simulink model "PMSM_SMC_C"  (R2022b)
settings: Solver=ode23tb  StartTime=0.0  StopTime=1  FixedStep=Ts  RelTol=1e-4  EnableMultiTasking=on
InitFcn:
  | Ts = 10e-6;
  | 
  | R = 2.875;
  | Ld = 8.2e-3;
  | Lq = 8.2e-3;
  | Pn = 4;
  | flux = 0.175;
  | alpha1=15;
  | alpha2=9;
  | e=0.0005;
  | B = 0;
  | J = 0.003;
  | a=-(B/J);
  | b=(3*Pn*flux)/(2*J);
  | kq1=100;
  | kq2=80;
undefined symbols (not defined in the file): DiscIntNeverNeededParam, k1, k2
libraries: simulink x3, powerlib_extras x1, slpidlib x1, spsPermanentMagnetSynchronousMachineLib x1, spsUniversalBridgeLib x1, spsDCVoltageSourceLib x1, sps_lib x1
settings Model: Creator=SUN  LastModifiedBy=hl
settings SolverCC: ZeroCrossControl=DisableAll  AlgebraicLoopSolver=TrustRegion
settings DataIOCC: LimitDataPoints=on  SaveFormat=Array  SignalLoggingSaveFormat=ModelDataLogs  ReturnWorkspaceOutputs=off
settings OptimizationCC: ExpressionDepthLimit=2147483647  InitFltsAndDblsToZero=on  LifeSpan=inf
settings DebuggingCC: UnderspecifiedInitializationDetection=Classic  MergeDetectMultiDrivingBlocksExec=none  SolverPrmCheckMsg=warning  FcnCallInpInsideContextMsg=warning  UnconnectedInputMsg=warning  UnconnectedOutputMsg=warning  UnconnectedLineMsg=warning  StateNameClashWarn=warning  SFUnexpectedBacktrackingDiag=warning  SFNoUnconditionalDefaultTransitionDiag=warning  SFMachineParentedDataDiag=warning  ArithmeticOperatorsInVariantConditions=warning
settings HardwareCC: ProdBitPerPointer=32  ProdBitPerSizeT=32  ProdBitPerPtrDiffT=32  ProdLargestAtomicFloat=None  ProdIntDivRoundTo=Undefined  ProdEndianess=Unspecified  ProdWordSize=32  ProdHWDeviceType=32-bit Generic
settings ModelReferenceCC: EnableRefExpFcnMdlSchedulingChecks=on  PropagateSignalLabelsOutOfModel=off
settings SFSimCC: SimUseLocalCustomCode=off  CustomCodeUndefinedFunction=UseInterfaceOnly
settings RTWCC: RTWUseLocalCustomCode=off
settings CodeAppCC: StateflowObjectComments=on
settings GRTTargetCC: TargetLangStandard=C89/C90 (ANSI)  CombineOutputUpdateFcns=off  GRTInterface=on
settings ConfigComp: CovMetricSettings=dw  CovSaveCumulativeToWorkspaceVar=on  CovSaveSingleToWorkspaceVar=on  CovExternalEMLEnable=off  CovSFcnEnable=off
settings SimscapeCC: SimscapeNormalizeSystem=off

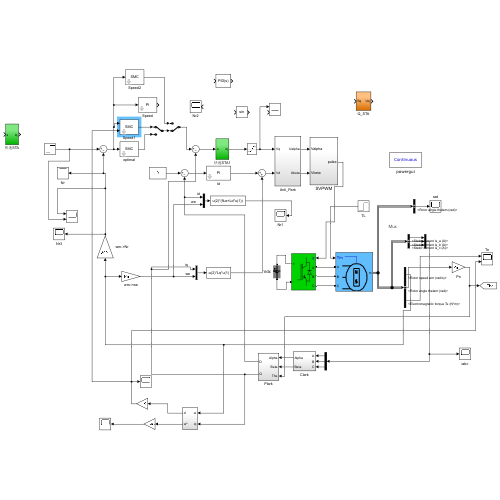
[thumbnail: Simulink's stored preview of the top-level diagram]
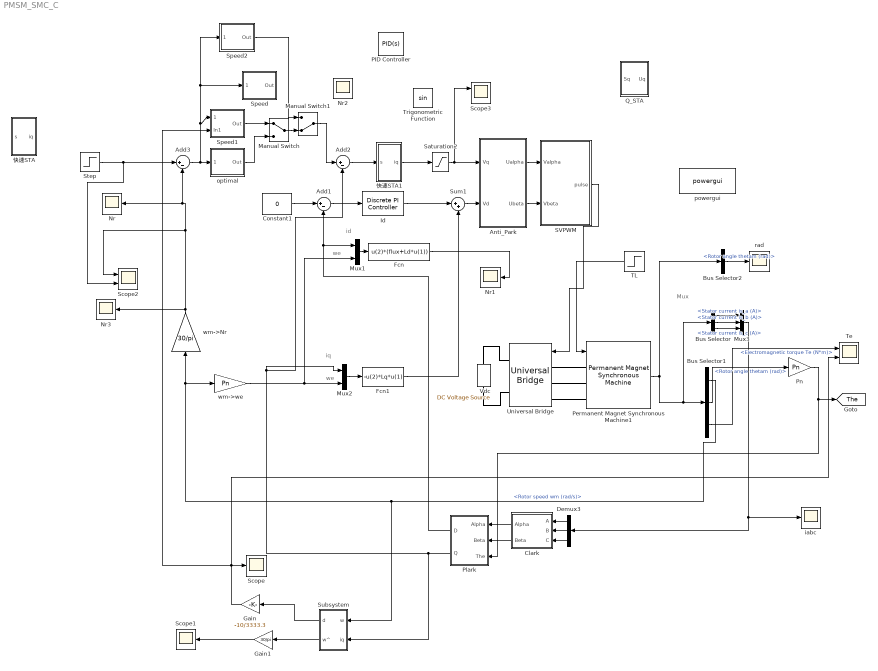
== system PMSM_SMC_C ==
  note: Mux
  note: iq
  note: we
  note: we
  note: id
  Add1 : Sum  Inputs=|+-
  Add2 : Sum  Inputs=|+-
  Add3 : Sum  Inputs=|+-
  Anti_Park : Subsystem
  Bus Selector : BusSelector  OutputSignals=Stator current is_a (A),Stator current is_b (A),Stator current is_c (A)
  Bus Selector1 : BusSelector  OutputSignals=Rotor speed wm (rad/s),Rotor angle thetam (rad),Electromagnetic torque Te (N*m)
  Bus Selector2 : BusSelector  OutputSignals=Rotor angle thetam (rad)
  Clark : Subsystem
  Constant1 : Constant  Value=0
  Demux3 : Demux  Outputs=3
  Fcn : Fcn  Expr=u(2)*(flux+Ld*u(1))
  Fcn1 : Fcn  Expr=-u(2)*Lq*u(1)
  Gain : Gain  Gain=-10/3333.3
  Gain1 : Gain  Gain=30/pi
  Id : powerlib_extras/Discrete  Control Blocks/Discrete PI Controller  Kp=Ld*2000  Ki=R*2000  Par_Limits=[311*0.9*sqrt(1/3) -311*0.9*sqrt(1/3)]  Init=0  Ts=Ts
  Manual Switch : ManualSwitch
  Manual Switch1 : ManualSwitch  CurrentSetting=0
  Mux1 : Mux  Inputs=2
  Mux2 : Mux  Inputs=2
  Mux3 : Mux  Inputs=3
  Nr{,1..3} (4 alike) : Scope
  PID Controller : slpidlib/PID Controller  Controller=PID  Form=Parallel  TimeDomain=Continuous-time  UseExternalTs=off  SampleTime=-1  IntegratorMethod=Forward Euler  FilterMethod=Forward Euler  ControllerParametersSource=internal  P=60  I=10  UseKiTs=off  D=0  N=100  UseFilter=on  TunerSelectOption=Transfer Function Based (PID Tuner App)  InitialConditionSource=internal  InitialConditionForIntegrator=0  InitialConditionForFilter=0  DifferentiatorICPrevScaledInput=0  ExternalReset=none  TrackingMode=off  Kt=1  LimitOutput=off  SatLimitsSource=internal  UpperSaturationLimit=inf  LowerSaturationLimit=-inf  LinearizeAsGain=on  AntiWindupMode=none  Kb=1  LimitIntegrator=off  UpperIntegratorSaturationLimit=inf  LowerIntegratorSaturationLimit=-inf  POutMin=[]  POutMax=[]  IOutMin=[]  IOutMax=[]  DOutMin=[]  DOutMax=[]  NOutMin=[]  NOutMax=[]  SumOutMin=[]  SumOutMax=[]  SaturationOutMin=[]  SaturationOutMax=[]  PParamMin=[]  PParamMax=[]  IParamMin=[]  IParamMax=[]  DParamMin=[]  DParamMax=[]  NParamMin=[]  NParamMax=[]  KbParamMin=[]  KbParamMax=[]  KtParamMin=[]  KtParamMax=[]  KbOutMin=[]  KbOutMax=[]  KtOutMin=[]  KtOutMax=[]  IntegratorOutMin=[]  IntegratorOutMax=[]  FilterOutMin=[]  FilterOutMax=[]  SumI1OutMin=[]  SumI1OutMax=[]  SumI2OutMin=[]  SumI2OutMax=[]  SumI3OutMin=[]  SumI3OutMax=[]  SumI4OutMin=[]  SumI4OutMax=[]  SumDOutMin=[]  SumDOutMax=[]  DifferentiatorOutMin=[]  DifferentiatorOutMax=[]  FilterDiffOutCoefMin=[]  FilterDiffOutCoefMax=[]  ReciprocalOutMin=[]  ReciprocalOutMax=[]  SumDenOutMin=[]  SumDenOutMax=[]  SumNumOutMin=[]  SumNumOutMax=[]  DivideOutMin=[]  DivideOutMax=[]  UdiffTsProdOutMin=[]  UdiffTsProdOutMax=[]  NTsProdOutMin=[]  NTsProdOutMax=[]  UintegralTsProdOutMin=[]  UintegralTsProdOutMax=[]  UngainTsProdOutMin=[]  UngainTsProdOutMax=[]  ClampingZeroOutDataTypeStr=Inherit: Inherit via back propagation  ClampingZeroOutMin=[]  ClampingZeroOutMax=[]  FilterDenConstantOutDataTypeStr=Inherit: Inherit via back propagation  FilterDenConstantOutMin=[]  FilterDenConstantOutMax=[]  PCopyOutDataTypeStr=Inherit: Inherit via back propagation  PCopyOutMin=[]  PCopyOutMax=[]  NCopyOutDataTypeStr=Inherit: Inherit via back propagation  NCopyOutMin=[]  NCopyOutMax=[]  IntegratorContinuousStateAttributes=''  IntegratorStateMustResolveToSignalObject=off  IntegratorRTWStateStorageClass=Auto  FilterContinuousStateAttributes=''  FilterStateMustResolveToSignalObject=off  FilterRTWStateStorageClass=Auto  ParallelPVariant=InternalParameters  IdealPVariant=Disabled  IVariant=InternalParameters  DVariant=InternalParameters  IntegratorVariant=Continuous  SatVariant=Disabled  AWVariant=Passthrough  PCopyVariant=Disabled  TRVariant=Disabled  FdbkBlocksVariant=Forward  IdealPFdbkVariant=Disabled  SatFdbkVariant=Disabled  DerivativeFilterVariant=ContFilter  NVariant=InternalParameters  NCopyVariant=Disabled  FilterICVariant=InternalICsFilter  IntegratorICVariant=InternalICs  ExternalResetVariant=Disabled  TRSumVariant=Passthrough  SumFdbkVariant=Disabled  SumVariant=Sum_PID  TsampFilterVariant=InternalTs  TsampNgainVariant=Passthrough  TsampIntegralVariant=Passthrough  ExternalSaturationOutDataTypeStr=Inherit: Same as second input
  Permanent Magnet Synchronous Machine1 : spsPermanentMagnetSynchronousMachineLib/Permanent Magnet Synchronous Machine  NbPhases=3  FluxDistribution=Sinusoidal  RotorType=Salient-pole  MechanicalLoad=Torque Tm  PresetModel=No  ShowDetailedParameters=on  MeasurementBus=off  Resistance=2.875  Inductance=8.5e-3  dqInductances=[8.5e-3,8.5e-3]  La=0.000835  MachineConstant=Flux linkage established by magnets (V.s)  Flux=0.175  VoltageCst=126.966  TorqueCst=1.05  Flat=120  Mechanical=[0.003 0.008 4 0]  PolePairs=3  InitialConditions=[0,0, 0,0]  InitialConditions5ph=[0 0 0 0 0 0]  RefAngle=Aligned with phase A axis (original Park)  IterativeDiscreteModel=Trapezoidal non iterative  TsBlock=-1  TsPowergui=0
  Plark : Subsystem
  Pn : Gain  Gain=Pn
  Q_STA : Subsystem
  SVPWM : Subsystem
  Saturation2 : Saturate  UpperLimit=380  LowerLimit=-400  SampleTime=Ts
  Scope : Scope
  Scope1 : Scope
  Scope2 : Scope  NumInputPorts=2
  Scope3 : Scope  NumInputPorts=2
  Speed : Subsystem  AncestorBlock=|  DialogController=POWERSYS.PowerSysDialog  mask(Discrete PI Controller){Kpw=0.14, Kiw=0.14*50, Ba=0.013, Par_Limits=[30 -30], Init=0, Ts=Ts}
      | powerlib_extras/Discrete 
      | Control Blocks/Discrete
      | PI Controller
      mask prompts: Kpw "Proportional gain (Kp):"; Kiw "Integral gain (Ki):"; Ba "feedback gain (Ba)"; Par_Limits "Output limits: [ Upper   Lower ]"; Init "Output initial value:"; Ts "Sample time:"
      mask help: This block implements a discrete PI controller.
      mask init:
      | UpperLimit=Par_Limits(1);
      | LowerLimit=Par_Limits(2);
      | power_initmask();
      settings: LibrarySourceBlock=|
      | powerlib_extras/Discrete
      | Control Blocks/Discrete
      | PI Controller
      mask Help: This block is part of a subset of blocks in the Extras library that does not have documentation associated with it, other than the block mask description.
      mask Display: disp('PI');
  Speed1 : Subsystem  AncestorBlock=|  DialogController=POWERSYS.PowerSysDialog  mask(Discrete PI Controller){C=600, Mu=200, q=300, Par_Limits=[30 -30], Init=0, Ts=Ts}
      | powerlib_extras/Discrete 
      | Control Blocks/Discrete
      | PI Controller
      mask prompts: C "Gain (c):"; Mu "Gain (Mu):"; q "Gain (q)"; Par_Limits "Output limits: [ Upper   Lower ]"; Init "Output initial value:"; Ts "Sample time:"
      mask help: This block implements a discrete PI controller.
      mask init:
      | UpperLimit=Par_Limits(1);
      | LowerLimit=Par_Limits(2);
      | power_initmask();
      settings: LibrarySourceBlock=|
      | powerlib_extras/Discrete
      | Control Blocks/Discrete
      | PI Controller
      mask Help: This block is part of a subset of blocks in the Extras library that does not have documentation associated with it, other than the block mask description.
      mask Display: disp('SMC');
  Speed2 : Subsystem  AncestorBlock=|  DialogController=POWERSYS.PowerSysDialog  mask(Discrete PI Controller){C=50, Mu=500, q=1000, Par_Limits=[30 -30], Init=0, Ts=Ts}
      | powerlib_extras/Discrete 
      | Control Blocks/Discrete
      | PI Controller
      mask prompts: C "Gain (c):"; Mu "Gain (Mu):"; q "Gain (q)"; Par_Limits "Output limits: [ Upper   Lower ]"; Init "Output initial value:"; Ts "Sample time:"
      mask help: This block implements a discrete PI controller.
      mask init:
      | UpperLimit=Par_Limits(1);
      | LowerLimit=Par_Limits(2);
      | power_initmask();
      settings: LibrarySourceBlock=|
      | powerlib_extras/Discrete
      | Control Blocks/Discrete
      | PI Controller
      mask Help: This block is part of a subset of blocks in the Extras library that does not have documentation associated with it, other than the block mask description.
      mask Display: disp('SMC');
  Step : Step  Time=0.6  Before=500  After=1000  SampleTime=0
  Subsystem : Subsystem
  Sum1 : Sum  Inputs=|++
  TL : Step  Time=0.3  After=10  SampleTime=0
  Te : Scope  NumInputPorts=2
  Trigonometric Function : Trigonometry
  Universal Bridge : spsUniversalBridgeLib/Universal Bridge  Arms=3  SnubberResistance=1e5  SnubberCapacitance=inf  Device=IGBT / Diodes  Ron=1e-3  Lon=0  ForwardVoltages="[  0  0  ]"  ForwardVoltage=0  GTOparameters=[ 10e-6 , 20e-6 ]  IGBTparameters=[ 1e-6 , 2e-6 ]  Measurements=None  Measurements_2=None  converterType=Rectifier
  Vdc : spsDCVoltageSourceLib/DC Voltage Source  Amplitude=311  Measurements=None
  iabc : Scope
  optimal : Subsystem  AncestorBlock=|  DialogController=POWERSYS.PowerSysDialog  mask(Discrete PI Controller){C=500, Mu=200, q=300, Par_Limits=[30 -30], Init=0, Ts=Ts}
      | powerlib_extras/Discrete 
      | Control Blocks/Discrete
      | PI Controller
      mask prompts: C "Gain (c):"; Mu "Gain (Mu):"; q "Gain (q)"; Par_Limits "Output limits: [ Upper   Lower ]"; Init "Output initial value:"; Ts "Sample time:"
      mask help: This block implements a discrete PI controller.
      mask init:
      | UpperLimit=Par_Limits(1);
      | LowerLimit=Par_Limits(2);
      | power_initmask();
      settings: LibrarySourceBlock=|
      | powerlib_extras/Discrete
      | Control Blocks/Discrete
      | PI Controller
      mask Help: This block is part of a subset of blocks in the Extras library that does not have documentation associated with it, other than the block mask description.
      mask Display: disp('SMC');
  powergui : sps_lib/powergui  SimulationMode=Continuous  SampleTime=Ts  frequency=60  Iterations=50  frequencyindice=0  Pbase=100e6  ErrMax=1e-4  UnitsV=kV  UnitsW=MW  buscounter=0  FunctionMessages=off  echomessages=off  EnableUseOfTLC=off  CurrentSourceSwitches=on  DisableSnubberDevices=off  DisableRonSwitches=off  DisableVfSwitches=off  DisplayEquations=off  AutomaticDiscreteSolvers=off  SolverType=Tustin/Backward Euler (TBE)  Interpol=off  ExternalGateDelay=off  methode=off  Ts=0  x0status=blocks  SPID=off  SwTol=0  HookPort=off  NonlinearTolerance=1e-4  nMaxIteration=100  ContinueOnMaxIteration=off  RestoreLinks=warning  ResistiveCurrentMeasurement=off  Frange=[0:2:500]  Ylog=off  Xlog=on  ShowGrid=off  save=off  variable=ZData  structure=0  ZoomFFT=on  StartTime=0.0  cycles=1  DisplayStyle=1  fundamental=60  FreqAxis=off  MaxFrequency=1000  frequencyindicesteady=1  RmsSteady=1  display=off
  rad : Scope
  wm->Nr : Gain  Gain=30/pi
  wm->we : Gain  Gain=Pn
  快速STA : Subsystem
  快速STA1 : Subsystem
  tag scope: The=global
  wires:
  TL/1 -> Permanent Magnet Synchronous Machine1/1
  Add3/1 -> Speed1/1(Error), Speed2/1(Error), Speed/1(Error), optimal/1(Error)
  Fcn1/1 -> Sum1/2
  Constant1/1 -> Add1/1
  wm->Nr/1 -> Scope2/1, Add3/2, Nr/1, Nr3/1
  wm->we/1 -> Mux2/2, Mux1/2
  Mux1/1 -> Fcn/1
  Mux2/1 -> Fcn1/1
  Sum1/1 -> Anti_Park/2(Vd)
  Pn/1 -> Plark/3(The), [The]
  SVPWM/1(pulse) -> Universal Bridge/1
  Mux3/1 -> iabc/1, Demux3/1
  Anti_Park/1(Ualpha) -> SVPWM/1(Valpha)
  Anti_Park/2(Ubeta) -> SVPWM/2(Vbeta)
  Clark/1(Alpha) -> Plark/1(Alpha)
  Demux3/1 -> Clark/1(A)
  Demux3/2 -> Clark/2(B)
  Demux3/3 -> Clark/3(C)
  Clark/2(Beta) -> Plark/2(Beta)
  Plark/1(D) -> Mux1/1, Add1/2
  Plark/2(Q) -> Subsystem/2(iq), Mux2/1, Add2/2
  Speed1/1(Out) -> Manual Switch/1
  optimal/1(Out) -> Manual Switch/2
  Manual Switch/1 -> Manual Switch1/2
  Bus Selector/1 -> Mux3/1  "<Stator current is_a (A)>"
  Bus Selector/3 -> Mux3/3  "<Stator current is_c (A)>"
  Bus Selector/2 -> Mux3/2  "<Stator current is_b (A)>"
  Permanent Magnet Synchronous Machine1/1 -> Bus Selector/1, Bus Selector1/1, Bus Selector2/1
  Bus Selector1/3 -> Te/1  "<Electromagnetic torque Te (N*m)>"
  Bus Selector1/2 -> Pn/1  "<Rotor angle thetam (rad)>"
  Bus Selector1/1 -> Subsystem/1(w), wm->we/1, wm->Nr/1  "<Rotor speed wm (rad/s)>"
  Bus Selector2/1 -> rad/1  "<Rotor angle thetam (rad)>"
  Subsystem/2(w^) -> Gain1/1
  Gain1/1 -> Scope1/1
  Subsystem/1(d) -> Gain/1
  Gain/1 -> Scope/1, Speed1/2(In1), Te/2
  Id/1 -> Sum1/1
  Add1/1 -> Id/1
  Step/1 -> Scope2/2, Add3/1
  Saturation2/1 -> Anti_Park/1(Vq), Scope3/1
  Manual Switch1/1 -> Add2/1
  Fcn/1 -> Nr1/1
  Speed2/1(Out) -> Manual Switch1/1
  Add2/1 -> 快速STA1/1(s)
  快速STA1/1(iq) -> Saturation2/1
  connections:
  Universal Bridge/RConn1 -- Vdc/RConn1
  Permanent Magnet Synchronous Machine1/LConn3 -- Universal Bridge/LConn3
  Permanent Magnet Synchronous Machine1/LConn2 -- Universal Bridge/LConn2
  Universal Bridge/RConn2 -- Vdc/LConn1
  Permanent Magnet Synchronous Machine1/LConn1 -- Universal Bridge/LConn1

== system PMSM_SMC_C/Anti_Park ==
  Vq : Inport
  Vd : Inport  Port=2
  Fcn : Fcn  Expr=cos(u[1])*u[2]-sin(u[1])*u[3]
  Fcn1 : Fcn  Expr=sin(u[1])*u[2]+cos(u[1])*u[3]
  Mux1 : Mux  Inputs=3
  Ualpha : Outport  VectorParamsAs1DForOutWhenUnconnected=off
  Ubeta : Outport  Port=2  VectorParamsAs1DForOutWhenUnconnected=off
  wires:
  Fcn1/1 -> Ubeta/1
  Fcn/1 -> Ualpha/1
  Mux1/1 -> Fcn/1, Fcn1/1
  Vd/1 -> Mux1/2
  Vq/1 -> Mux1/3
  [The] -> Mux1/1

== system PMSM_SMC_C/Clark ==
  A : Inport
  B : Inport  Port=2
  C : Inport  Port=3
  Mux : Mux  Inputs=3
  alpha : Fcn  Expr=(u(1)-0.5*(u(2)+u(3)))*2/3
  beta : Fcn  Expr=sqrt(3)/2*(u(2)-u(3))*2/3
  Alpha : Outport  VectorParamsAs1DForOutWhenUnconnected=off
  Beta : Outport  Port=2  VectorParamsAs1DForOutWhenUnconnected=off
  wires:
  alpha/1 -> Alpha/1
  B/1 -> Mux/2
  C/1 -> Mux/3
  A/1 -> Mux/1
  Mux/1 -> beta/1, alpha/1
  beta/1 -> Beta/1

== system PMSM_SMC_C/Plark ==
  Alpha : Inport
  Beta : Inport  Port=2
  The : Inport  Port=3
  Mux : Mux  Inputs=3
  d : Fcn  Expr=u(1)*cos(u(3))+u(2)*sin(u(3))
  q : Fcn  Expr=-u(1)*sin(u(3))+u(2)*cos(u(3))
  D : Outport  VectorParamsAs1DForOutWhenUnconnected=off
  Q : Outport  Port=2  VectorParamsAs1DForOutWhenUnconnected=off
  wires:
  d/1 -> D/1
  Beta/1 -> Mux/2
  The/1 -> Mux/3
  Alpha/1 -> Mux/1
  Mux/1 -> q/1, d/1
  q/1 -> Q/1

== system PMSM_SMC_C/Q_STA ==
  Sq : Inport
  Abs : Abs  SaturateOnIntegerOverflow=off
  Add : Sum
  Constant : Constant  Value=0.5
  Discrete-Time Integrator : DiscreteIntegrator  ICPrevOutput=DiscIntNeverNeededParam  ICPrevScaledInput=DiscIntNeverNeededParam
  Gain : Gain  Gain=kq1
  Gain1 : Gain  Gain=kq2
  Math Function : Math  Operator=pow  SignedPower=on
  Product : Product
  Sign : Signum
  Uq : Outport
  wires:
  Add/1 -> Uq/1
  Gain1/1 -> Discrete-Time Integrator/1
  Discrete-Time Integrator/1 -> Add/2
  Gain/1 -> Add/1
  Sq/1 -> Sign/1, Abs/1
  Product/1 -> Gain/1
  Sign/1 -> Gain1/1, Product/2
  Constant/1 -> Math Function/2
  Math Function/1 -> Product/1
  Abs/1 -> Math Function/1

== system PMSM_SMC_C/SVPWM ==
  Valpha : Inport
  Vbeta : Inport  Port=2
  PWM : Subsystem
  Repeating Sequence : simulink/Sources/Repeating Sequence  rep_seq_t=[0 0.00005 0.0001]  rep_seq_y=[0 0.00005 0]
  Sector Caculate : Subsystem
  T1T1 Caculate : Subsystem
  Tcm Caculate : Subsystem
  Tpwm : Constant  Value=0.0001
  Vdc : Constant  Value=311
  XYZ Caculate : Subsystem
  pulse : Outport  VectorParamsAs1DForOutWhenUnconnected=off
  wires:
  PWM/1(PWM) -> pulse/1
  Repeating Sequence/1 -> PWM/1(In)
  Vbeta/1 -> XYZ Caculate/2(Ubeta), Sector Caculate/2(Ubeta)
  T1T1 Caculate/1(T1) -> Tcm Caculate/2(T1)
  Valpha/1 -> XYZ Caculate/1(Ualpha), Sector Caculate/1(Ualpha)
  T1T1 Caculate/2(T2) -> Tcm Caculate/3(T2)
  Sector Caculate/1("N ") -> Tcm Caculate/1(N), T1T1 Caculate/1(N)
  XYZ Caculate/1(XYZ) -> T1T1 Caculate/2(XYZ)
  Tpwm/1 -> XYZ Caculate/3(Ts), Tcm Caculate/4(Tpwm), T1T1 Caculate/3(Tpwm)
  Vdc/1 -> XYZ Caculate/4(Udc)
  Tcm Caculate/1(Tcm1 Tcm2 Tcm3) -> PWM/2(Tcm123)

== system PMSM_SMC_C/Speed ==
  note: Discrete PID Controller
  note: Pierre Giroux, Gilbert Sybille
      | Power System Simulation Laboratory
      | IREQ, Hydro-Quebc
  Error : Inport  SampleTime=Ts
  Discrete-Time Integrator : DiscreteIntegrator  InitialCondition=Init  SampleTime=Ts  LimitOutput=on  UpperSaturationLimit=UpperLimit  LowerSaturationLimit=LowerLimit  ICPrevOutput=DiscIntNeverNeededParam  ICPrevScaledInput=DiscIntNeverNeededParam
  Kp1 : Gain  Gain=Ba  SaturateOnIntegerOverflow=on  SampleTime=Ts  OutDataTypeStr=Inherit: Same as input  ParamDataTypeStr=Inherit: Same as input
  Kp4 : Gain  Gain=Kpw  SaturateOnIntegerOverflow=on  SampleTime=Ts  OutDataTypeStr=Inherit: Same as input  ParamDataTypeStr=Inherit: Same as input
  Kp5 : Gain  Gain=Kiw  SaturateOnIntegerOverflow=on  SampleTime=Ts  OutDataTypeStr=Inherit: Same as input  ParamDataTypeStr=Inherit: Same as input
  Saturation2 : Saturate  UpperLimit=UpperLimit  LowerLimit=LowerLimit  SampleTime=Ts
  Sum6 : Sum  Inputs=++-  InputSameDT=on  SaturateOnIntegerOverflow=on  SampleTime=Ts  OutDataTypeStr=Inherit: Same as first input
  Zero-Order Hold : ZeroOrderHold  SampleTime=Ts
  Out : Outport  SampleTime=Ts  InitialOutput=0  VectorParamsAs1DForOutWhenUnconnected=off
  wires:
  Error/1 -> Kp1/1, Kp5/1, Kp4/1
  Zero-Order Hold/1 -> Sum6/1
  Saturation2/1 -> Out/1
  Discrete-Time Integrator/1 -> Sum6/2
  Kp4/1 -> Zero-Order Hold/1
  Kp5/1 -> Discrete-Time Integrator/1
  Sum6/1 -> Saturation2/1
  Kp1/1 -> Sum6/3

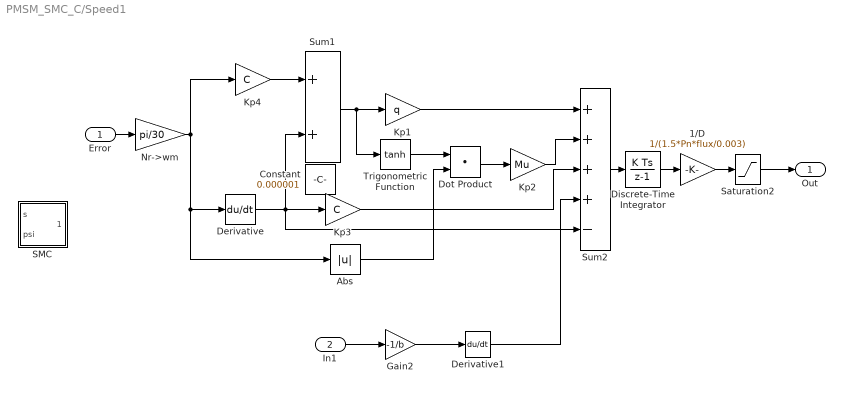
== system PMSM_SMC_C/Speed1 ==
  Error : Inport  SampleTime=Ts
  In1 : Inport  Port=2
  1/D : Gain  Gain=1/(1.5*Pn*flux/0.003)  SaturateOnIntegerOverflow=on  SampleTime=Ts  OutDataTypeStr=Inherit: Same as input  ParamDataTypeStr=Inherit: Same as input
  Abs : Abs  SaturateOnIntegerOverflow=off
  Constant : Constant  Value=0.000001
  Derivative : Derivative
  Derivative1 : Derivative
  Discrete-Time Integrator : DiscreteIntegrator  InitialCondition=0.001  SampleTime=Ts  ICPrevOutput=DiscIntNeverNeededParam  ICPrevScaledInput=DiscIntNeverNeededParam
  Dot Product : DotProduct  OutDataTypeStr=Inherit: Inherit via internal rule
  Gain2 : Gain  Gain=-1/b
  Kp1 : Gain  Gain=q  SaturateOnIntegerOverflow=on  SampleTime=Ts  OutDataTypeStr=Inherit: Same as input  ParamDataTypeStr=Inherit: Same as input
  Kp2 : Gain  Gain=Mu  SaturateOnIntegerOverflow=on  SampleTime=Ts  OutDataTypeStr=Inherit: Same as input  ParamDataTypeStr=Inherit: Same as input
  Kp3 : Gain  Gain=C  SaturateOnIntegerOverflow=on  SampleTime=Ts  OutDataTypeStr=Inherit: Same as input  ParamDataTypeStr=Inherit: Same as input
  Kp4 : Gain  Gain=C  SaturateOnIntegerOverflow=on  SampleTime=Ts  OutDataTypeStr=Inherit: Same as input  ParamDataTypeStr=Inherit: Same as input
  Nr->wm : Gain  Gain=pi/30  SaturateOnIntegerOverflow=on  SampleTime=Ts  OutDataTypeStr=Inherit: Same as input  ParamDataTypeStr=Inherit: Same as input
  SMC : MATLAB Function  TreatAsAtomicUnit=on
  Saturation2 : Saturate  UpperLimit=UpperLimit  LowerLimit=LowerLimit  SampleTime=Ts
  Sum1 : Sum  InputSameDT=on  SaturateOnIntegerOverflow=on  SampleTime=Ts  OutDataTypeStr=Inherit: Same as first input
  Sum2 : Sum  Inputs=++++-  InputSameDT=on  SaturateOnIntegerOverflow=on  SampleTime=Ts  OutDataTypeStr=Inherit: Same as first input
  Trigonometric Function : Trigonometry  Operator=tanh
  Out : Outport  SampleTime=Ts  InitialOutput=0  VectorParamsAs1DForOutWhenUnconnected=off
  wires:
  Kp4/1 -> Sum1/1
  Saturation2/1 -> Out/1
  Error/1 -> Nr->wm/1
  Kp1/1 -> Sum2/1
  Sum1/1 -> Trigonometric Function/1, Kp1/1
  Kp2/1 -> Sum2/2
  Kp3/1 -> Sum2/3
  Nr->wm/1 -> Kp4/1, Abs/1, Derivative/1
  Derivative/1 -> Sum2/5, Sum1/2, Kp3/1
  Sum2/1 -> Discrete-Time Integrator/1
  1/D/1 -> Saturation2/1
  Discrete-Time Integrator/1 -> 1/D/1
  Dot Product/1 -> Kp2/1
  Abs/1 -> Dot Product/2
  In1/1 -> Gain2/1
  Gain2/1 -> Derivative1/1
  Derivative1/1 -> Sum2/4
  Trigonometric Function/1 -> Dot Product/1

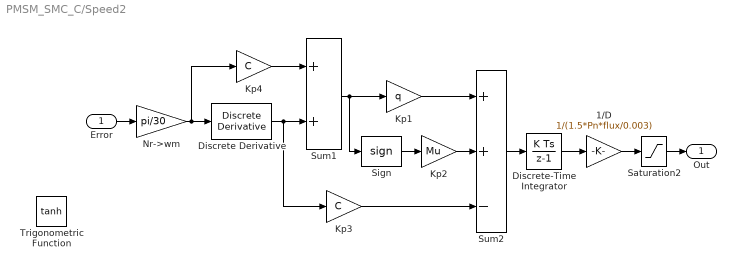
== system PMSM_SMC_C/Speed2 ==
  Error : Inport  SampleTime=Ts
  1/D : Gain  Gain=1/(1.5*Pn*flux/0.003)  SaturateOnIntegerOverflow=on  SampleTime=Ts  OutDataTypeStr=Inherit: Same as input  ParamDataTypeStr=Inherit: Same as input
  Discrete Derivative : simulink/Discrete/Discrete Derivative  gainval=1.0  ICPrevScaledInput=0.0  OutMin=[]  OutMax=[]  OutDataType=fixdt(1, 16)  OutScaling=2^-10  DoSatur=off
  Discrete-Time Integrator : DiscreteIntegrator  InitialCondition=0.001  SampleTime=Ts  ICPrevOutput=DiscIntNeverNeededParam  ICPrevScaledInput=DiscIntNeverNeededParam
  Kp1 : Gain  Gain=q  SaturateOnIntegerOverflow=on  SampleTime=Ts  OutDataTypeStr=Inherit: Same as input  ParamDataTypeStr=Inherit: Same as input
  Kp2 : Gain  Gain=Mu  SaturateOnIntegerOverflow=on  SampleTime=Ts  OutDataTypeStr=Inherit: Same as input  ParamDataTypeStr=Inherit: Same as input
  Kp3 : Gain  Gain=C  SaturateOnIntegerOverflow=on  SampleTime=Ts  OutDataTypeStr=Inherit: Same as input  ParamDataTypeStr=Inherit: Same as input
  Kp4 : Gain  Gain=C  SaturateOnIntegerOverflow=on  SampleTime=Ts  OutDataTypeStr=Inherit: Same as input  ParamDataTypeStr=Inherit: Same as input
  Nr->wm : Gain  Gain=pi/30  SaturateOnIntegerOverflow=on  SampleTime=Ts  OutDataTypeStr=Inherit: Same as input  ParamDataTypeStr=Inherit: Same as input
  Saturation2 : Saturate  UpperLimit=UpperLimit  LowerLimit=LowerLimit  SampleTime=Ts
  Sign : Signum
  Sum1 : Sum  InputSameDT=on  SaturateOnIntegerOverflow=on  SampleTime=Ts  OutDataTypeStr=Inherit: Same as first input
  Sum2 : Sum  Inputs=++-  InputSameDT=on  SaturateOnIntegerOverflow=on  SampleTime=Ts  OutDataTypeStr=Inherit: Same as first input
  Trigonometric Function : Trigonometry  Operator=tanh  OutputSignalType=real
  Out : Outport  SampleTime=Ts  InitialOutput=0
  wires:
  Kp4/1 -> Sum1/1
  Saturation2/1 -> Out/1
  Discrete Derivative/1 -> Kp3/1, Sum1/2
  Sum2/1 -> Discrete-Time Integrator/1
  Error/1 -> Nr->wm/1
  Kp1/1 -> Sum2/1
  Sum1/1 -> Kp1/1, Sign/1
  Kp2/1 -> Sum2/2
  Kp3/1 -> Sum2/3
  1/D/1 -> Saturation2/1
  Discrete-Time Integrator/1 -> 1/D/1
  Nr->wm/1 -> Discrete Derivative/1, Kp4/1
  Sign/1 -> Kp2/1

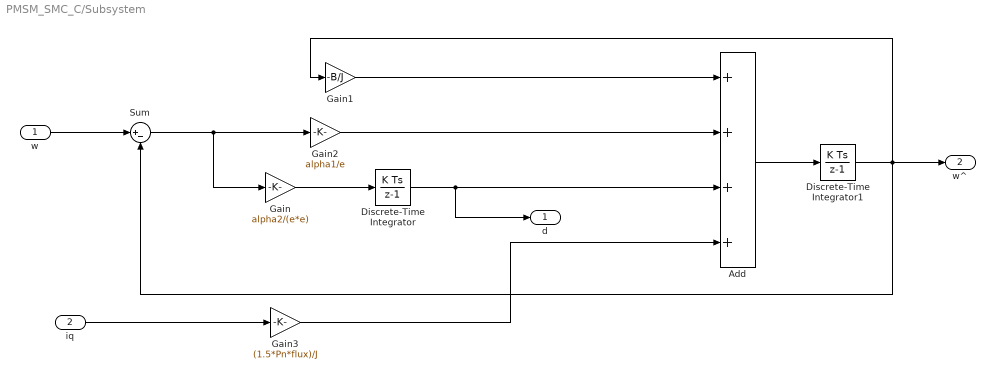
== system PMSM_SMC_C/Subsystem ==
  w : Inport
  iq : Inport  Port=2
  Add : Sum  Inputs=++++
  Discrete-Time Integrator : DiscreteIntegrator  SampleTime=Ts  ICPrevOutput=DiscIntNeverNeededParam  ICPrevScaledInput=DiscIntNeverNeededParam
  Discrete-Time Integrator1 : DiscreteIntegrator  SampleTime=Ts  ICPrevOutput=DiscIntNeverNeededParam  ICPrevScaledInput=DiscIntNeverNeededParam
  Gain : Gain  Gain=alpha2/(e*e)
  Gain1 : Gain  Gain=-B/J
  Gain2 : Gain  Gain=alpha1/e
  Gain3 : Gain  Gain=(1.5*Pn*flux)/J
  Sum : Sum  Inputs=|+-
  d : Outport  VectorParamsAs1DForOutWhenUnconnected=off
  w^ : Outport  Port=2  VectorParamsAs1DForOutWhenUnconnected=off
  wires:
  Gain1/1 -> Add/1
  Discrete-Time Integrator/1 -> Add/3, d/1
  Gain/1 -> Discrete-Time Integrator/1
  Add/1 -> Discrete-Time Integrator1/1
  Gain2/1 -> Add/2
  Discrete-Time Integrator1/1 -> Sum/2, Gain1/1, w^/1
  Gain3/1 -> Add/4
  iq/1 -> Gain3/1
  Sum/1 -> Gain2/1, Gain/1
  w/1 -> Sum/1

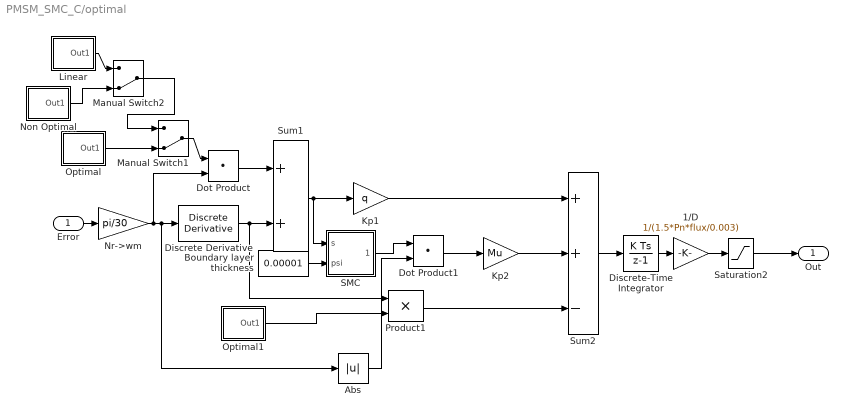
== system PMSM_SMC_C/optimal ==
  Error : Inport  SampleTime=Ts
  1/D : Gain  Gain=1/(1.5*Pn*flux/0.003)  SaturateOnIntegerOverflow=on  SampleTime=Ts  OutDataTypeStr=Inherit: Same as input  ParamDataTypeStr=Inherit: Same as input
  Abs : Abs  SaturateOnIntegerOverflow=off
  Boundary layer thickness : Constant  Value=0.00001
  Discrete Derivative : simulink/Discrete/Discrete Derivative  gainval=1.0  ICPrevScaledInput=0.0  OutMin=[]  OutMax=[]  OutDataType=fixdt(1, 16)  OutScaling=2^-10  DoSatur=off
  Discrete-Time Integrator : DiscreteIntegrator  InitialCondition=0.001  SampleTime=Ts  ICPrevOutput=DiscIntNeverNeededParam  ICPrevScaledInput=DiscIntNeverNeededParam
  Dot Product : DotProduct  OutDataTypeStr=Inherit: Inherit via internal rule
  Dot Product1 : DotProduct  OutDataTypeStr=Inherit: Inherit via internal rule
  Kp1 : Gain  Gain=q  SaturateOnIntegerOverflow=on  SampleTime=Ts  OutDataTypeStr=Inherit: Same as input  ParamDataTypeStr=Inherit: Same as input
  Kp2 : Gain  Gain=Mu  SaturateOnIntegerOverflow=on  SampleTime=Ts  OutDataTypeStr=Inherit: Same as input  ParamDataTypeStr=Inherit: Same as input
  Linear : Subsystem
  Manual Switch1 : ManualSwitch  CurrentSetting=0
  Manual Switch2 : ManualSwitch  CurrentSetting=0
  "Non Optimal " : Subsystem
  Nr->wm : Gain  Gain=pi/30  SaturateOnIntegerOverflow=on  SampleTime=Ts  OutDataTypeStr=Inherit: Same as input  ParamDataTypeStr=Inherit: Same as input
  Optimal : Subsystem
  Optimal1 : Subsystem
  Product1 : Product
  SMC : MATLAB Function  TreatAsAtomicUnit=on
  Saturation2 : Saturate  UpperLimit=UpperLimit  LowerLimit=LowerLimit  SampleTime=Ts
  Sum1 : Sum  InputSameDT=on  SaturateOnIntegerOverflow=on  SampleTime=Ts  OutDataTypeStr=Inherit: Same as first input
  Sum2 : Sum  Inputs=++-  InputSameDT=on  SaturateOnIntegerOverflow=on  SampleTime=Ts  OutDataTypeStr=Inherit: Same as first input
  Out : Outport  SampleTime=Ts  InitialOutput=0  VectorParamsAs1DForOutWhenUnconnected=off
  wires:
  Saturation2/1 -> Out/1
  Sum2/1 -> Discrete-Time Integrator/1
  Error/1 -> Nr->wm/1
  Kp1/1 -> Sum2/1
  Sum1/1 -> SMC/1(s), Kp1/1
  Kp2/1 -> Sum2/2
  1/D/1 -> Saturation2/1
  Discrete-Time Integrator/1 -> 1/D/1
  Boundary layer thickness/1 -> SMC/2(psi)
  Dot Product/1 -> Sum1/1
  Discrete Derivative/1 -> Product1/1, Sum1/2
  Manual Switch1/1 -> Dot Product/1
  Manual Switch2/1 -> Manual Switch1/1
  "Non Optimal "/1(Out1) -> Manual Switch2/2
  Linear/1(Out1) -> Manual Switch2/1
  Optimal/1(Out1) -> Manual Switch1/2
  Product1/1 -> Sum2/3
  Optimal1/1(Out1) -> Product1/2
  Nr->wm/1 -> Dot Product/2, Abs/1, Discrete Derivative/1
  SMC/1(output) -> Dot Product1/1
  Abs/1 -> Dot Product1/2
  Dot Product1/1 -> Kp2/1

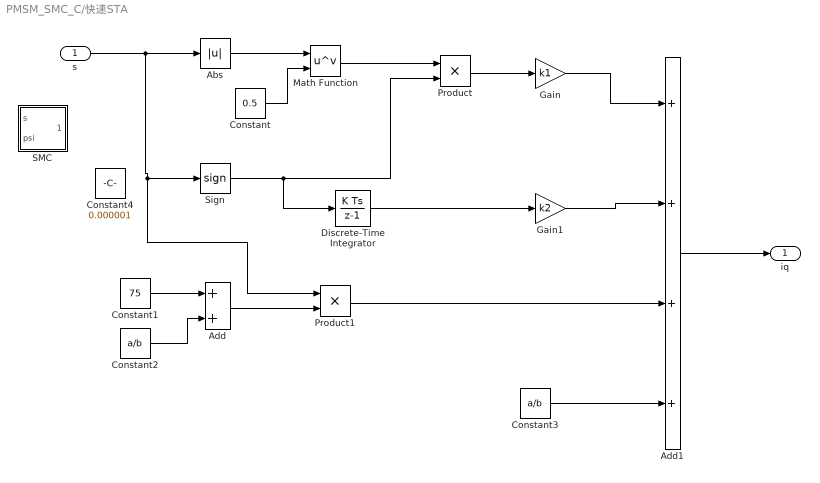
== system PMSM_SMC_C/快速STA ==
  s : Inport
  Abs : Abs  SaturateOnIntegerOverflow=off
  Add : Sum
  Add1 : Sum  Inputs=++++
  Constant : Constant  Value=0.5
  Constant1 : Constant  Value=75
  Constant2 : Constant  Value=a/b
  Constant3 : Constant  Value=a/b
  Constant4 : Constant  Value=0.000001
  Discrete-Time Integrator : DiscreteIntegrator  ICPrevOutput=DiscIntNeverNeededParam  ICPrevScaledInput=DiscIntNeverNeededParam
  Gain : Gain  Gain=k1
  Gain1 : Gain  Gain=k2
  Math Function : Math  Operator=pow  SignedPower=on
  Product : Product
  Product1 : Product
  SMC : MATLAB Function  TreatAsAtomicUnit=on
  Sign : Signum
  iq : Outport
  wires:
  Abs/1 -> Math Function/1
  Discrete-Time Integrator/1 -> Gain1/1
  Constant/1 -> Math Function/2
  s/1 -> Sign/1, Product1/1, Abs/1
  Math Function/1 -> Product/1
  Gain1/1 -> Add1/2
  Add1/1 -> iq/1
  Gain/1 -> Add1/1
  Product/1 -> Gain/1
  Constant1/1 -> Add/1
  Constant2/1 -> Add/2
  Add/1 -> Product1/2
  Product1/1 -> Add1/3
  Constant3/1 -> Add1/4
  Sign/1 -> Product/2, Discrete-Time Integrator/1

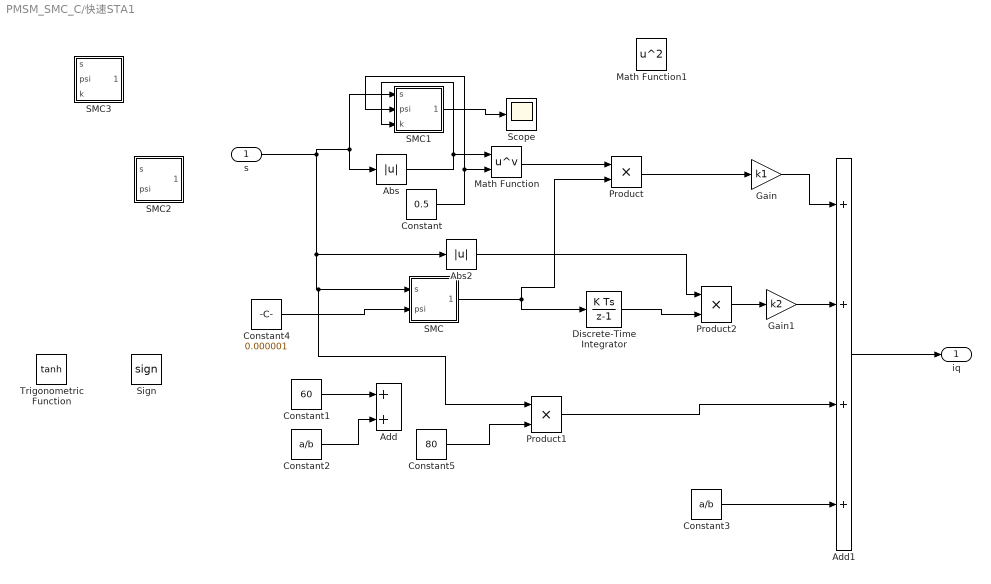
== system PMSM_SMC_C/快速STA1 ==
  s : Inport
  Abs : Abs  SaturateOnIntegerOverflow=off
  Abs2 : Abs  SaturateOnIntegerOverflow=off
  Add : Sum
  Add1 : Sum  Inputs=++++
  Constant : Constant  Value=0.5
  Constant1 : Constant  Value=60
  Constant2 : Constant  Value=a/b
  Constant3 : Constant  Value=a/b
  Constant4 : Constant  Value=0.000001
  Constant5 : Constant  Value=80
  Discrete-Time Integrator : DiscreteIntegrator  ICPrevOutput=DiscIntNeverNeededParam  ICPrevScaledInput=DiscIntNeverNeededParam
  Gain : Gain  Gain=k1
  Gain1 : Gain  Gain=k2
  Math Function : Math  Operator=pow  SignedPower=on
  Math Function1 : Math  Operator=square  SignedPower=on
  Product : Product
  Product1 : Product
  Product2 : Product
  SMC : MATLAB Function  TreatAsAtomicUnit=on
  SMC1 : MATLAB Function  TreatAsAtomicUnit=on
  SMC2 : MATLAB Function  TreatAsAtomicUnit=on
  SMC3 : MATLAB Function  TreatAsAtomicUnit=on
  Scope : Scope
  Sign : Signum
  Trigonometric Function : Trigonometry  Operator=tanh
  iq : Outport
  wires:
  s/1 -> Abs/1, SMC1/1(s), Abs2/1, Product1/1, SMC/1(s)
  Gain1/1 -> Add1/2
  Add1/1 -> iq/1
  Gain/1 -> Add1/1
  Constant1/1 -> Add/1
  Constant2/1 -> Add/2
  Product1/1 -> Add1/3
  Constant3/1 -> Add1/4
  Abs/1 -> Math Function/1, SMC1/3(k)
  Constant/1 -> Math Function/2, SMC1/2(psi)
  SMC1/1(output) -> Scope/1
  Product/1 -> Gain/1
  Math Function/1 -> Product/1
  SMC/1(output) -> Product/2, Discrete-Time Integrator/1
  Constant4/1 -> SMC/2(psi)
  Constant5/1 -> Product1/2
  Product2/1 -> Gain1/1
  Discrete-Time Integrator/1 -> Product2/2
  Abs2/1 -> Product2/1

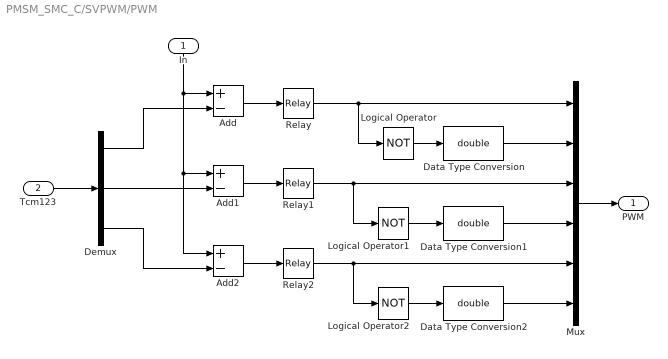
== system PMSM_SMC_C/SVPWM/PWM ==
  In : Inport
  Tcm123 : Inport  Port=2
  Add : Sum  Inputs=+-
  Add1 : Sum  Inputs=+-
  Add2 : Sum  Inputs=+-
  Data Type Conversion : DataTypeConversion  OutDataTypeStr=double  SaturateOnIntegerOverflow=off  RndMeth=Floor
  Data Type Conversion1 : DataTypeConversion  OutDataTypeStr=double  SaturateOnIntegerOverflow=off  RndMeth=Floor
  Data Type Conversion2 : DataTypeConversion  OutDataTypeStr=double  SaturateOnIntegerOverflow=off  RndMeth=Floor
  Demux : Demux  Outputs=3
  Logical Operator : Logic  Operator=NOT  AllPortsSameDT=off  OutDataTypeStr=boolean
  Logical Operator1 : Logic  Operator=NOT  AllPortsSameDT=off  OutDataTypeStr=boolean
  Logical Operator2 : Logic  Operator=NOT  AllPortsSameDT=off  OutDataTypeStr=boolean
  Mux : Mux  Inputs=6
  Relay : Relay  OffSwitchValue=-eps
  Relay1 : Relay  OffSwitchValue=-eps
  Relay2 : Relay  OffSwitchValue=-eps
  PWM : Outport  VectorParamsAs1DForOutWhenUnconnected=off
  wires:
  Demux/3 -> Add2/2
  Demux/2 -> Add1/2
  Demux/1 -> Add/2
  Relay2/1 -> Mux/5, Logical Operator2/1
  Relay1/1 -> Mux/3, Logical Operator1/1
  Relay/1 -> Logical Operator/1, Mux/1
  Mux/1 -> PWM/1
  Data Type Conversion/1 -> Mux/2
  Data Type Conversion1/1 -> Mux/4
  Data Type Conversion2/1 -> Mux/6
  Logical Operator2/1 -> Data Type Conversion2/1
  Logical Operator1/1 -> Data Type Conversion1/1
  Logical Operator/1 -> Data Type Conversion/1
  Add1/1 -> Relay1/1
  Add2/1 -> Relay2/1
  Add/1 -> Relay/1
  In/1 -> Add/1, Add2/1, Add1/1
  Tcm123/1 -> Demux/1

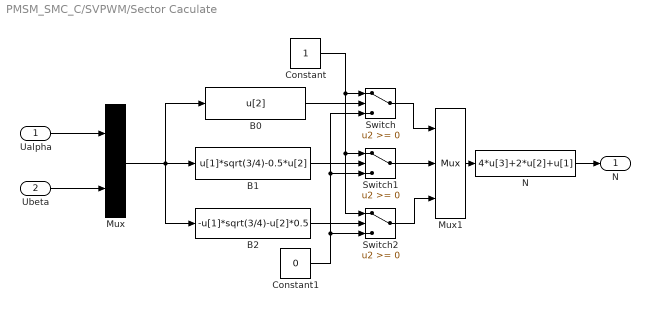
== system PMSM_SMC_C/SVPWM/Sector Caculate ==
  Ualpha : Inport
  Ubeta : Inport  Port=2
  B0 : Fcn  Expr=u[2]
  B1 : Fcn  Expr=u[1]*sqrt(3/4)-0.5*u[2]
  B2 : Fcn  Expr=-u[1]*sqrt(3/4)-u[2]*0.5
  Constant : Constant
  Constant1 : Constant  Value=0
  Mux : Mux  Inputs=2
  Mux1 : Mux  Inputs=3
  N : Fcn  Expr=4*u[3]+2*u[2]+u[1]
  Switch : Switch  SaturateOnIntegerOverflow=off  InputSameDT=off
  Switch1 : Switch  SaturateOnIntegerOverflow=off  InputSameDT=off
  Switch2 : Switch  SaturateOnIntegerOverflow=off  InputSameDT=off
  "N " : Outport  VectorParamsAs1DForOutWhenUnconnected=off
  wires:
  Switch2/1 -> Mux1/3
  Switch/1 -> Mux1/1
  Ualpha/1 -> Mux/1
  Ubeta/1 -> Mux/2
  Mux/1 -> B2/1, B1/1, B0/1
  B0/1 -> Switch/2
  B1/1 -> Switch1/2
  B2/1 -> Switch2/2
  Constant/1 -> Switch/1, Switch2/1, Switch1/1
  Constant1/1 -> Switch/3, Switch1/3, Switch2/3
  Switch1/1 -> Mux1/2
  Mux1/1 -> N/1
  N/1 -> "N "/1

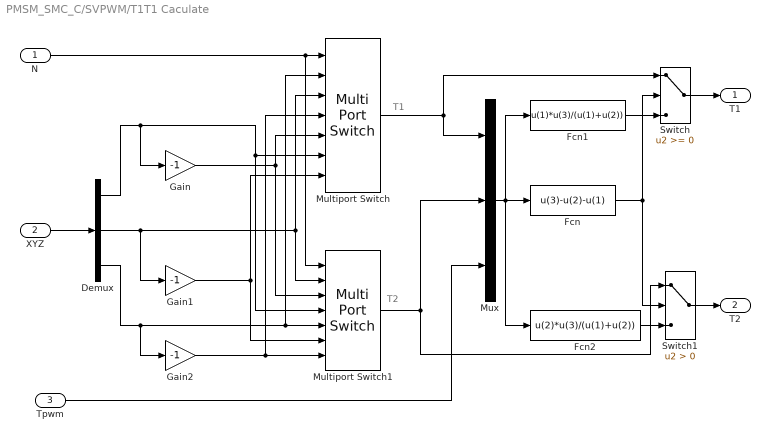
== system PMSM_SMC_C/SVPWM/T1T1 Caculate ==
  note: T1
  note: T2
  N : Inport
  XYZ : Inport  Port=2
  Tpwm : Inport  Port=3
  Demux : Demux  Outputs=3
  Fcn : Fcn  Expr=u(3)-u(2)-u(1)
  Fcn1 : Fcn  Expr=u(1)*u(3)/(u(1)+u(2))
  Fcn2 : Fcn  Expr=u(2)*u(3)/(u(1)+u(2))
  Gain : Gain  Gain=-1
  Gain1 : Gain  Gain=-1
  Gain2 : Gain  Gain=-1
  Multiport Switch : MultiPortSwitch  Inputs=6  SaturateOnIntegerOverflow=off  InputSameDT=off
  Multiport Switch1 : MultiPortSwitch  Inputs=6  SaturateOnIntegerOverflow=off  InputSameDT=off
  Mux : Mux  Inputs=3
  Switch : Switch  SaturateOnIntegerOverflow=off  InputSameDT=off
  Switch1 : Switch  Criteria=u2 > Threshold  SaturateOnIntegerOverflow=off  InputSameDT=off
  T1 : Outport  VectorParamsAs1DForOutWhenUnconnected=off
  T2 : Outport  Port=2  VectorParamsAs1DForOutWhenUnconnected=off
  wires:
  Tpwm/1 -> Mux/3
  XYZ/1 -> Demux/1
  Switch1/1 -> T2/1
  Switch/1 -> T1/1
  Fcn2/1 -> Switch1/3
  Fcn1/1 -> Switch/3
  Fcn/1 -> Switch/2, Switch1/2
  Mux/1 -> Fcn1/1, Fcn/1, Fcn2/1
  Multiport Switch/1 -> Switch/1, Mux/1
  Multiport Switch1/1 -> Switch1/1, Mux/2
  N/1 -> Multiport Switch/1, Multiport Switch1/1
  Demux/2 -> Multiport Switch/3, Multiport Switch1/2, Gain1/1
  Demux/3 -> Multiport Switch1/5, Multiport Switch/2, Gain2/1
  Demux/1 -> Multiport Switch/6, Multiport Switch1/4, Gain/1
  Gain/1 -> Multiport Switch1/3, Multiport Switch/5
  Gain2/1 -> Multiport Switch/4, Multiport Switch1/7
  Gain1/1 -> Multiport Switch1/6, Multiport Switch/7

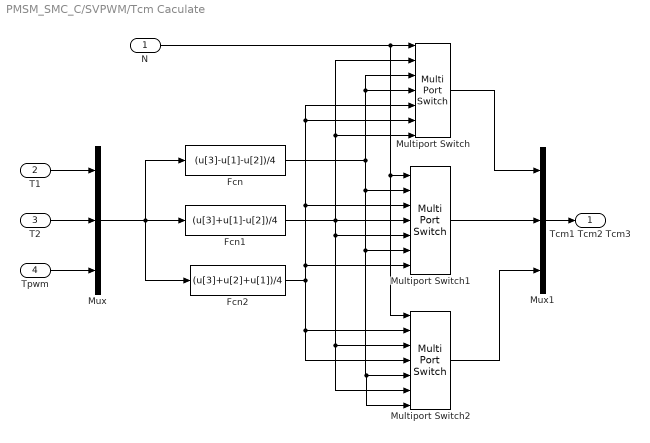
== system PMSM_SMC_C/SVPWM/Tcm Caculate ==
  N : Inport
  T1 : Inport  Port=2
  T2 : Inport  Port=3
  Tpwm : Inport  Port=4
  Fcn : Fcn  Expr=(u[3]-u[1]-u[2])/4
  Fcn1 : Fcn  Expr=(u[3]+u[1]-u[2])/4
  Fcn2 : Fcn  Expr=(u[3]+u[2]+u[1])/4
  Multiport Switch : MultiPortSwitch  Inputs=6  SaturateOnIntegerOverflow=off  InputSameDT=off
  Multiport Switch1 : MultiPortSwitch  Inputs=6  SaturateOnIntegerOverflow=off  InputSameDT=off
  Multiport Switch2 : MultiPortSwitch  Inputs=6  SaturateOnIntegerOverflow=off  InputSameDT=off
  Mux : Mux  Inputs=3
  Mux1 : Mux  Inputs=3
  Tcm1 Tcm2 Tcm3 : Outport  VectorParamsAs1DForOutWhenUnconnected=off
  wires:
  Mux/1 -> Fcn2/1, Fcn/1, Fcn1/1
  Tpwm/1 -> Mux/3
  T2/1 -> Mux/2
  T1/1 -> Mux/1
  Multiport Switch2/1 -> Mux1/3
  Multiport Switch1/1 -> Mux1/2
  Multiport Switch/1 -> Mux1/1
  Mux1/1 -> Tcm1 Tcm2 Tcm3/1
  Fcn/1 -> Multiport Switch/3, Multiport Switch/4, Multiport Switch1/6, Multiport Switch2/5, Multiport Switch2/7, Multiport Switch1/2
  Fcn1/1 -> Multiport Switch1/5, Multiport Switch2/3, Multiport Switch2/6, Multiport Switch1/4, Multiport Switch/7, Multiport Switch/2
  Fcn2/1 -> Multiport Switch/5, Multiport Switch/6, Multiport Switch1/3, Multiport Switch1/7, Multiport Switch2/2, Multiport Switch2/4
  N/1 -> Multiport Switch2/1, Multiport Switch1/1, Multiport Switch/1

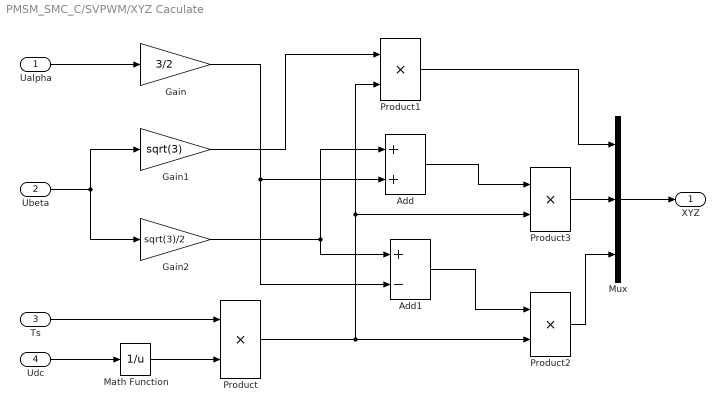
== system PMSM_SMC_C/SVPWM/XYZ Caculate ==
  Ualpha : Inport
  Ubeta : Inport  Port=2
  Ts : Inport  Port=3
  Udc : Inport  Port=4
  Add : Sum
  Add1 : Sum  Inputs=+-
  Gain : Gain  Gain=3/2
  Gain1 : Gain  Gain=sqrt(3)
  Gain2 : Gain  Gain=sqrt(3)/2
  Math Function : Math  Operator=reciprocal  SignedPower=on
  Mux : Mux  Inputs=3
  Product{,1..3} (4 alike) : Product  RndMeth=Zero
  XYZ : Outport  VectorParamsAs1DForOutWhenUnconnected=off
  wires:
  Mux/1 -> XYZ/1
  Product1/1 -> Mux/1
  Product3/1 -> Mux/2
  Product2/1 -> Mux/3
  Ualpha/1 -> Gain/1
  Ubeta/1 -> Gain2/1, Gain1/1
  Udc/1 -> Math Function/1
  Math Function/1 -> Product/2
  Ts/1 -> Product/1
  Gain1/1 -> Product1/1
  Product/1 -> Product2/2, Product1/2, Product3/2
  Gain/1 -> Add1/2, Add/2
  Gain2/1 -> Add/1, Add1/1
  Add1/1 -> Product2/1
  Add/1 -> Product3/1

== system PMSM_SMC_C/optimal/Linear ==
  Clock : Clock
  Saturation : Saturate  UpperLimit=20
  system1 : Fcn  Expr=(36.07*u(1)) + 2
  Out1 : Outport  VectorParamsAs1DForOutWhenUnconnected=off
  wires:
  Clock/1 -> system1/1
  system1/1 -> Saturation/1
  Saturation/1 -> Out1/1

== system PMSM_SMC_C/optimal/Non Optimal  ==
  note: good: (20-2)/(1+exp(-4*u(1)+6)) + 2
  Clock : Clock
  system1 : Fcn  Expr=(20-2)/(1+exp(-22*u(1)+6)) + 2
  Out1 : Outport  VectorParamsAs1DForOutWhenUnconnected=off
  wires:
  Clock/1 -> system1/1
  system1/1 -> Out1/1

== system PMSM_SMC_C/optimal/Optimal ==
  Clock : Clock
  Constant  20 : Constant  Value=40
  If : If  IfExpression=u1 == 40  ShowElse=off
  If Action Subsystem : Subsystem  TreatAsAtomicUnit=on
  Rounding Function : Rounding  Operator=fix
  Scope : Scope  NumInputPorts=3
  Switch : Switch  Threshold=-2  SaturateOnIntegerOverflow=off  InputSameDT=off
  system1 : Fcn  Expr=(2+exp(2*u(1)))/(2-exp(2*u(1)))
  Out1 : Outport  VectorParamsAs1DForOutWhenUnconnected=off
  wires:
  Switch/1 -> Out1/1, Scope/3
  Clock/1 -> system1/1
  system1/1 -> Rounding Function/1, Switch/1, Scope/1
  If Action Subsystem/1(Out1) -> Switch/2, Scope/2
  Constant  20/1 -> Switch/3
  Rounding Function/1 -> If/1
  If/1 -> If Action Subsystem/Action

== system PMSM_SMC_C/optimal/Optimal1 ==
  Clock : Clock
  Constant  20 : Constant  Value=40
  If : If  IfExpression=u1 == 40  ShowElse=off
  If Action Subsystem : Subsystem  TreatAsAtomicUnit=on
  Rounding Function : Rounding  Operator=fix
  Switch : Switch  Threshold=-2  SaturateOnIntegerOverflow=off  InputSameDT=off
  system1 : Fcn  Expr=(2+exp(2*u(1)))/(2-exp(2*u(1)))
  Out1 : Outport  VectorParamsAs1DForOutWhenUnconnected=off
  wires:
  Switch/1 -> Out1/1
  Clock/1 -> system1/1
  system1/1 -> Rounding Function/1, Switch/1
  If Action Subsystem/1(Out1) -> Switch/2
  Constant  20/1 -> Switch/3
  Rounding Function/1 -> If/1
  If/1 -> If Action Subsystem/Action

== system PMSM_SMC_C/optimal/Optimal/If Action Subsystem ==
  Action Port : ActionPort  ActionPortLabel=if(u1 == 40)
  Constant  20 : Constant  Value=-3
  Out1 : Outport  VectorParamsAs1DForOutWhenUnconnected=off
  wires:
  Constant  20/1 -> Out1/1

== system PMSM_SMC_C/optimal/Optimal1/If Action Subsystem ==
  Action Port : ActionPort  ActionPortLabel=if(u1 == 40)
  Constant  20 : Constant  Value=-3
  Out1 : Outport  VectorParamsAs1DForOutWhenUnconnected=off
  wires:
  Constant  20/1 -> Out1/1

== matlab function PMSM_SMC_C/Speed1/SMC ==
  data: s input; output output; psi input
function output = smc(s, psi)
%#codegen  psi=1 即没有控制边界


    
        
    if (s > psi)    
        sat_s = 1;
    else if(abs(s)<psi)
        sat_s = s/psi;
        else
            sat_s=-1;
        end
    end
    
    output = sat_s;

end

== matlab function PMSM_SMC_C/optimal/SMC ==
  data: s input; output output; psi input
function output = smc(s, psi)
%#codegen  psi=1 即没有控制边界


    
        
    if (abs(s) > psi)    
        sat_s = sign(s);
    else
        sat_s = s/psi;
    end
    
    output = sat_s;

end

== matlab function PMSM_SMC_C/快速STA/SMC ==
  data: s input; output output; psi input
function output = smc(s, psi)
%#codegen  psi=1 即没有控制边界


    
        
    if (s > psi)    
        sat_s = 1;
    else if(abs(s)<psi)
        sat_s = s/psi;
        else
            sat_s=-1;
        end
    end
    
    output = sat_s;

end

== matlab function PMSM_SMC_C/快速STA1/SMC ==
  data: s input; output output; psi input
function output = smc(s, psi)
%#codegen  psi=1 即没有控制边界


    
        
    if (s > psi)    
        sat_s = 1;
    else if(abs(s)<psi)
        sat_s = s/psi;
        else
            sat_s=-1;
        end
    end
    
    output = sat_s;

end

== matlab function PMSM_SMC_C/快速STA1/SMC1 ==
  data: s input; output output; psi input; k input
function output = smc(s, psi,k)
%#codegen  psi=1 即没有控制边界
output = (0.5-exp(-(psi*s)))/(0.5+exp(-(psi*s)));
if(output>0)
    output = output;
else
    output = -output;
end           
 output = k^output;
    end

== matlab function PMSM_SMC_C/快速STA1/SMC2 ==
  data: s input; output output; psi input
function output = smc(s, psi)
%#codegen  psi=1 即没有控制边界
  if (s > psi)    
        sat_s = 1;
    else if(abs(s)<psi)
        sat_s = s/psi;
        else
            sat_s=-1;
        end
    end
    
    output = sat_s;

    end

== matlab function PMSM_SMC_C/快速STA1/SMC3 ==
  data: s input; output output; psi input; k input
function output = smc(s, psi,k)
%#codegen  psi=1 即没有控制边界
output = (1-exp(-(psi*s)))/(1+exp(-(psi*s)));
if(output>0)
    output = output;
else
    output = -output;
end           
 output = k^output;
    end
